simulink model "MOT_CTRL_MOT_FUN_003"  (R2025a)
settings: Solver=FixedStepAuto  StartTime=0.0  StopTime=10  FixedStep=1e-4  RelTol=1e-3
libraries: simulink x1
settings Model: DataDictionary=DcMotor.sldd  Creator=tecnicomcbti  LastModifiedBy=tecnicomcbti
settings SolverCC: ConcurrentTasks=on  PositivePriorityOrder=on
settings OptimizationCC: BlockReduction=off  OptimizeBlockIOStorage=off  ZeroExternalMemoryAtStartup=off  ZeroInternalMemoryAtStartup=off
settings DebuggingCC: AlgebraicLoopMsg=none  TasksWithSamePriorityMsg=none
settings RTWCC: Toolchain=Simulink Real-Time Toolchain  BuildConfiguration=Faster Runs  CodeExecutionProfiling=on  TargetLang=C++
settings GRTTargetCC: TargetLangStandard=C++03 (ISO)  CodeInterfacePackaging=C++ class  SubcomponentCodeInterfacePackaging=C++ class

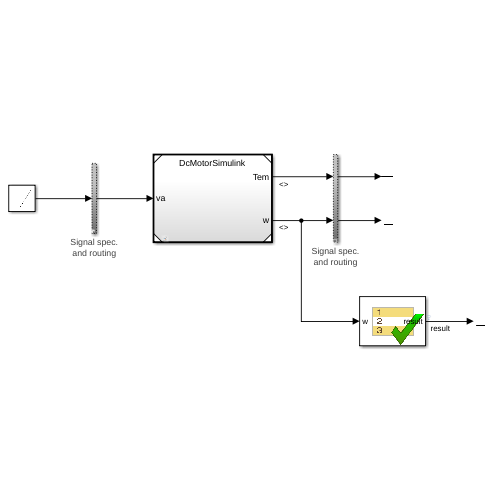
[thumbnail: Simulink's stored preview of the top-level diagram]
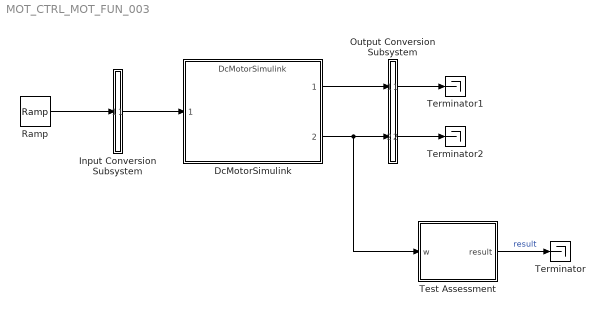
== system MOT_CTRL_MOT_FUN_003 ==
  DcMotorSimulink : ModelReference  ModelNameDialog=DcMotorSimulink  SimulationMode=Normal  ModelReferenceVersion=2.8
  Input Conversion Subsystem : Subsystem  Tag=__SLT_ICS__  Description=|
      | Signal spec.
      | and routing
      settings: AttributesFormatString=%<Description>
  Output Conversion Subsystem : Subsystem  Tag=__SLT_OCS__  Description=|
      | Signal spec.
      | and routing
      settings: AttributesFormatString=%<Description>
  Ramp : simulink/Sources/Ramp  slope=33  start=0  InitialOutput=0
  Terminator : Terminator
  Terminator1 : Terminator
  Terminator2 : Terminator
  Test Assessment : Test Sequence  TreatAsAtomicUnit=on
  wires:
  Input Conversion Subsystem/1(Outport_1) -> DcMotorSimulink/1
  DcMotorSimulink/1 -> Output Conversion Subsystem/1(Inport_1)
  DcMotorSimulink/2 -> Test Assessment/1(w), Output Conversion Subsystem/2(Inport_2)
  Test Assessment/1(result) -> Terminator/1  "result"
  Ramp/1 -> Input Conversion Subsystem/1(Inport_1)
  Output Conversion Subsystem/1(Outport_1) -> Terminator1/1
  Output Conversion Subsystem/2(Outport_2) -> Terminator2/1

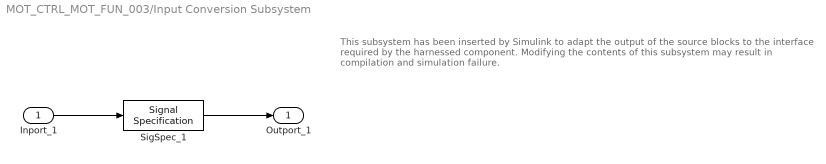
== system MOT_CTRL_MOT_FUN_003/Input Conversion Subsystem ==
  note: This subsystem has been inserted by Simulink to adapt the output of the source blocks to the interface required by the harnessed component.
      |  Modifying the contents of this subsystem may result in compilation and simulation failure.
  Inport_1 : Inport
  SigSpec_1 : SignalSpecification  OutDataTypeStr=double  Dimensions=[1]  SampleTime=[0, 0]
  Outport_1 : Outport
  wires:
  SigSpec_1/1 -> Outport_1/1
  Inport_1/1 -> SigSpec_1/1

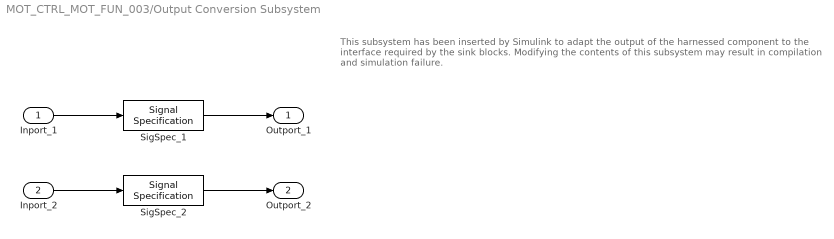
== system MOT_CTRL_MOT_FUN_003/Output Conversion Subsystem ==
  note: This subsystem has been inserted by Simulink to adapt the output of the harnessed component to the interface required by the sink blocks.
      |  Modifying the contents of this subsystem may result in compilation and simulation failure.
  Inport_1 : Inport
  Inport_2 : Inport  Port=2
  SigSpec_1 : SignalSpecification  OutDataTypeStr=double  Dimensions=[1]
  SigSpec_2 : SignalSpecification  OutDataTypeStr=double  Dimensions=[1]
  Outport_1 : Outport
  Outport_2 : Outport  Port=2
  wires:
  Inport_1/1 -> SigSpec_1/1
  SigSpec_1/1 -> Outport_1/1
  Inport_2/1 -> SigSpec_2/1
  SigSpec_2/1 -> Outport_2/1

== stateflow chart MOT_CTRL_MOT_FUN_003/Test Assessment ==
  state step_2
    if((w >= 0) && (w <= MAX_SPEED))
    result = true;
    else
    result = false;
    end
    settings: description=Se a entrada estiver entre 0 e 4500, a saída é verdadeira, se não, é falsa.
  (default) -> step_2
  data: w input; result output boolean; MAX_SPEED constant double =5100*pi/30
